simulink library "vco_snn"  (R2023b)
settings: Solver=VariableStepAuto  StartTime=0.0  StopTime=10.0  RelTol=1e-3
libraries: simulink_extras x166, spsSeriesRLCBranchLib x132, spsControlledVoltageSourceLib x126, $bdroot x33, fl_lib x18, msbPllFoundation x10, nesl_utility x9, spsVoltageMeasurementLib x8, simulink x6, spsGroundLib x5, eeGeneralControl x2
(part 1 of 2)
settings Model: Creator=saisanjeet  LastModifiedBy=saisanjeet

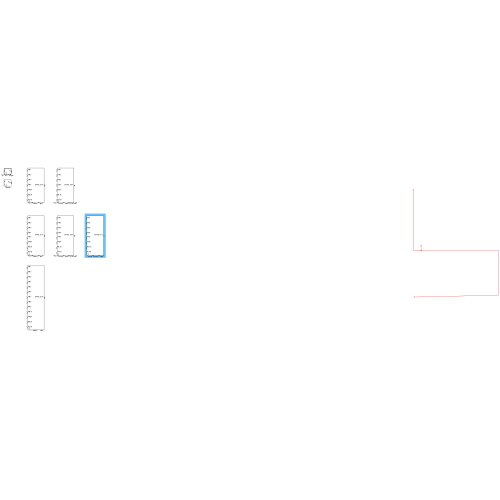
[thumbnail: Simulink's stored preview of the top-level diagram]
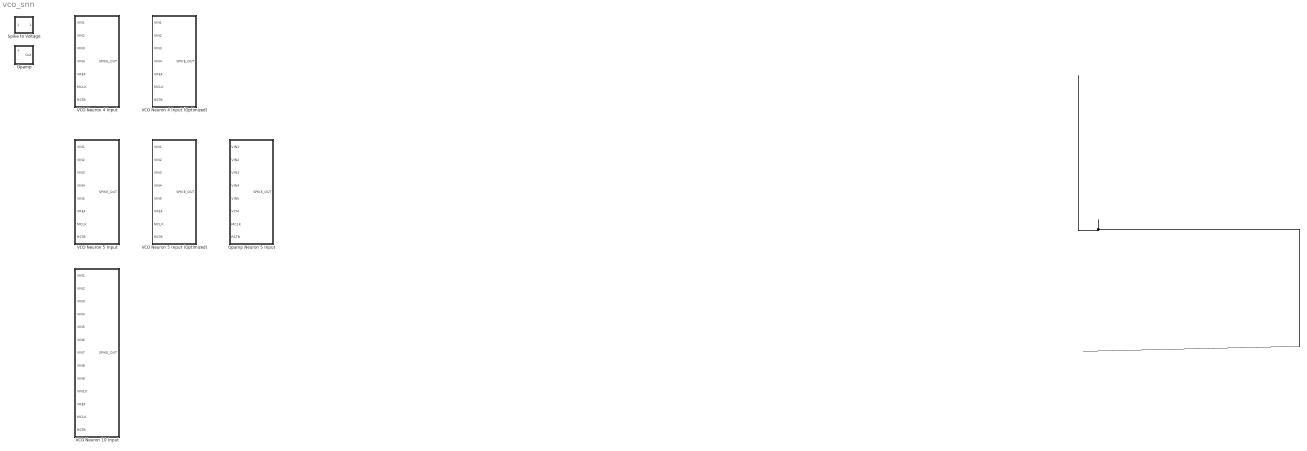
== system vco_snn ==
  Opamp : Subsystem  mask{Gain=1e3}
      mask prompts: Gain "Simulink:blkprm_prompts:GainGain"
      mask TypeOptions Gain: Gain1/Gain
      mask DialogControl Gain Prompt: Gain:
  Opamp Neuron 5 Input : Subsystem  mask{rf=25e3, cf=2e-12, vth=0.45, vcm=0.5, spike_amp=0.2, rin1=25e3, spike_sign1=+1, rin2=25e3, spike_sign2=+1, rin3=25e3, spike_sign3=+1, rin4=25e3, spike_sign4=+1, rin5=25e3, spike_sign5=+1}
      mask prompts: rf "Feedback Resistance (Ohms):"; cf "Feedback Capacitance (F):"; vth "Threshold Voltage (V):"; vcm "Common Mode (V):"; spike_amp "Spike Amplitude (V):"; rin1 "Input 1 Resistance (Ohms):"; spike_sign1 "Input 1 Sign:"; rin2 "Input 2 Resistance (Ohms):"; spike_sign2 "Input 2 Sign:"; rin3 "Input 3 Resistance (Ohms):"; spike_sign3 "Input 3 Sign:"; rin4 "Input 4 Resistance (Ohms):"; spike_sign4 "Input 4 Sign:"; rin5 "Input 5 Resistance (Ohms):"; spike_sign5 "Input 5 Sign:"
      mask TypeOptions rf: Resistor2/R
      mask TypeOptions cf: Capacitor/c
      mask TypeOptions vth:
      | Compare
      | To Constant/const
  Spike to Voltage : Subsystem  TreatAsAtomicUnit=on  mask{vcm=0.5, spike_amp=0.2, sign=+1}
      mask prompts: vcm "Common Mode Voltage (V):"; spike_amp "Spike Amplitude (V):"; sign "Spike Direction:"
      mask TypeOptions vcm: Add Constant/Bias
  VCO Neuron 10 Input : Subsystem  mask{kvco=10e6, center_freq=150e6, xor_res=50e3, vout_cap=1e-12, rf=25000, vth=0.45, vcm=0.5, spike_amp=0.2, rin1=25000, spike_sign1=+1, rin2=25000, spike_sign2=+1, rin3=25000, spike_sign3=+1, rin4=25000, spike_sign4=+1, rin5=25000, spike_sign5=+1, rin6=25000, spike_sign6=+1, rin7=25000, spike_sign7=+1, rin8=25000, spike_sign8=+1, rin9=25000, spike_sign9=+1, rin10=25000, spike_sign10=+1}
      mask prompts: kvco "Kvco (Hz/V):"; center_freq "Center Freq (Hz):"; xor_res "XNOR Resistance (Ohms):"; vout_cap "Output Capacitance (F):"; rf "Feedback Resistance (Ohms):"; vth "Threshold Voltage (V):"; vcm "Input Common Mode (V):"; spike_amp "Spike Amplitude (V):"; rin1 "Input 1 Resistance (Ohms):"; spike_sign1 "Input 1 Sign:"; rin2 "Input 2 Resistance (Ohms):"; spike_sign2 "Input 2 Sign:"; rin3 "Input 3 Resistance (Ohms):"; spike_sign3 "Input 3 Sign:"; rin4 "Input 4 Resistance (Ohms):"; spike_sign4 "Input 4 Sign:"; rin5 "Input 5 Resistance (Ohms):"; spike_sign5 "Input 5 Sign:"; rin6 "Input 6 Resistance (Ohms):"; spike_sign6 "Input 6 Sign:"; rin7 "Input 7 Resistance (Ohms):"; spike_sign7 "Input 7 Sign:"; rin8 "Input 8 Resistance (Ohms):"; spike_sign8 "Input 8 Sign:"; rin9 "Input 9 Resistance (Ohms):"; spike_sign9 "Input 9 Sign:"; rin10 "Input 10 Resistance (Ohms):"; spike_sign10 "Input 10 Sign:"
      mask TypeOptions vout_cap: cout/Capacitance
      mask TypeOptions rf: rf/Resistance
      mask TypeOptions vth: comp/const
  VCO Neuron 4 Input : Subsystem  mask{kvco=10e6, center_freq=150e6, xor_res=50e3, vout_cap=1e-12, rf=25000, vth=0.45, vcm=0.5, spike_amp=0.2, rin1=25000, spike_sign1=+1, rin2=25000, spike_sign2=+1, rin3=25000, spike_sign3=+1, rin4=25000, spike_sign4=+1}
      mask prompts: kvco "Kvco (Hz/V):"; center_freq "Center Freq (Hz):"; xor_res "XNOR Resistance (Ohms):"; vout_cap "Output Capacitance (F):"; rf "Feedback Resistance (Ohms):"; vth "Threshold Voltage (V):"; vcm "Input Common Mode (V):"; spike_amp "Spike Amplitude (V):"; rin1 "Input 1 Resistance (Ohms):"; spike_sign1 "Input 1 Sign:"; rin2 "Input 2 Resistance (Ohms):"; spike_sign2 "Input 2 Sign:"; rin3 "Input 3 Resistance (Ohms):"; spike_sign3 "Input 3 Sign:"; rin4 "Input 4 Resistance (Ohms):"; spike_sign4 "Input 4 Sign:"
      mask TypeOptions vout_cap: cout/Capacitance
      mask TypeOptions rf: rf/Resistance
      mask TypeOptions vth: comp/const
  VCO Neuron 4 Input (Optimized) : Subsystem  mask{kvco=10e6, center_freq=100e6, xor_tau=1.5625e-09, rf=25000, vth=0.45, vcm=0.5, spike_amp=0.2, rin1=25e3, spike_sign1=+1, rin2=25e3, spike_sign2=+1, rin3=25e3, spike_sign3=+1, rin4=25e3, spike_sign4=+1}
      mask prompts: kvco "Kvco (Hz/V):"; center_freq "Center Freq (Hz):"; xor_tau "XNOR Output Time Constant:"; rf "Feedback Resistance (Ohms):"; vth "Threshold Voltage (V):"; vcm "Input Common Mode (V):"; spike_amp "Spike Amplitude (V):"; rin1 "Input 1 Resistance (Ohms):"; spike_sign1 "Input 1 Sign:"; rin2 "Input 2 Resistance (Ohms):"; spike_sign2 "Input 2 Sign:"; rin3 "Input 3 Resistance (Ohms):"; spike_sign3 "Input 3 Sign:"; rin4 "Input 4 Resistance (Ohms):"; spike_sign4 "Input 4 Sign:"
      mask TypeOptions xor_tau: xor_lpf/T
      mask TypeOptions rf: rf/Resistance
      mask TypeOptions vth: comp/const
  VCO Neuron 5 Input : Subsystem  mask{kvco=10e6, center_freq=150e6, xor_res=50e3, vout_cap=1e-12, rf=25000, vth=0.45, vcm=0.5, spike_amp=0.2, rin1=25000, spike_sign1=+1, rin2=25000, spike_sign2=+1, rin3=25000, spike_sign3=+1, rin4=25000, spike_sign4=+1, rin5=25000, spike_sign5=+1}
      mask prompts: kvco "Kvco (Hz/V):"; center_freq "Center Freq (Hz):"; xor_res "XNOR Resistance (Ohms):"; vout_cap "Output Capacitance (F):"; rf "Feedback Resistance (Ohms):"; vth "Threshold Voltage (V):"; vcm "Input Common Mode (V):"; spike_amp "Spike Amplitude (V):"; rin1 "Input 1 Resistance (Ohms):"; spike_sign1 "Input 1 Sign:"; rin2 "Input 2 Resistance (Ohms):"; spike_sign2 "Input 2 Sign:"; rin3 "Input 3 Resistance (Ohms):"; spike_sign3 "Input 3 Sign:"; rin4 "Input 4 Resistance (Ohms):"; spike_sign4 "Input 4 Sign:"; rin5 "Input 5 Resistance (Ohms):"; spike_sign5 "Input 5 Sign:"
      mask TypeOptions vout_cap: cout/Capacitance
      mask TypeOptions rf: rf/Resistance
      mask TypeOptions vth: comp/const
  VCO Neuron 5 Input (Optimized) : Subsystem  mask{kvco=10e6, center_freq=120e6, xor_tau=1.5625e-09, rf=25000, vth=0.45, vcm=0.5, spike_amp=0.2, rin1=25000, spike_sign1=+1, rin2=25000, spike_sign2=+1, rin3=25000, spike_sign3=+1, rin4=25000, spike_sign4=+1, rin5=25000, spike_sign5=+1}
      mask prompts: kvco "Kvco (Hz/V):"; center_freq "Center Freq (Hz):"; xor_tau "XNOR Output Time Constant:"; rf "Feedback Resistance (Ohms):"; vth "Threshold Voltage (V):"; vcm "Input Common Mode (V):"; spike_amp "Spike Amplitude (V):"; rin1 "Input 1 Resistance (Ohms):"; spike_sign1 "Input 1 Sign:"; rin2 "Input 2 Resistance (Ohms):"; spike_sign2 "Input 2 Sign:"; rin3 "Input 3 Resistance (Ohms):"; spike_sign3 "Input 3 Sign:"; rin4 "Input 4 Resistance (Ohms):"; spike_sign4 "Input 4 Sign:"; rin5 "Input 5 Resistance (Ohms):"; spike_sign5 "Input 5 Sign:"
      mask TypeOptions xor_tau: xor_lpf/T
      mask TypeOptions rf: rf/Resistance
      mask TypeOptions vth: comp/const
  connections:
  ?
  ?

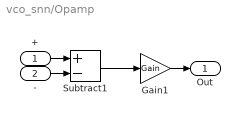
== system vco_snn/Opamp ==
  + : Inport
  - : Inport  Port=2
  Gain1 : Gain  Gain=Gain
  Subtract1 : Sum  Inputs=+-
  Out : Outport
  wires:
  -/1 -> Subtract1/2
  +/1 -> Subtract1/1
  Gain1/1 -> Out/1
  Subtract1/1 -> Gain1/1

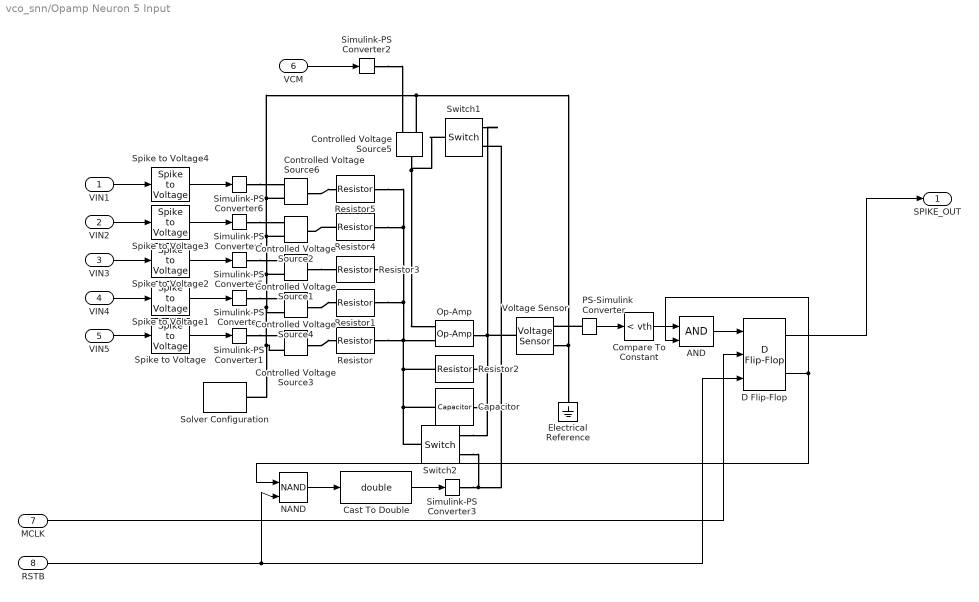
== system vco_snn/Opamp Neuron 5 Input ==
  VIN1 : Inport
  VIN2 : Inport  Port=2
  VIN3 : Inport  Port=3
  VIN4 : Inport  Port=4
  VIN5 : Inport  Port=5
  VCM : Inport  Port=6
  MCLK : Inport  Port=7
  RSTB : Inport  Port=8
  AND : Logic  IconShape=distinctive  AllPortsSameDT=off  OutDataTypeStr=boolean
  Capacitor : fl_lib/Electrical/Electrical Elements/Capacitor  c=cf F  r=1e-6 Ohm  g=0 1/Ohm  i_specify=off  i_priority=None  i=0 A  i_nominal_specify=off  i_nominal_unit=A  i_nominal_value=1  v_specify=on  v_priority=None  v=0 V  v_nominal_specify=off  v_nominal_unit=V  v_nominal_value=1  vc_specify=off  vc_priority=High  vc=0 V  vc_nominal_specify=off  vc_nominal_unit=V  vc_nominal_value=1
  Cast To Double : DataTypeConversion  OutDataTypeStr=double  SaturateOnIntegerOverflow=off  RndMeth=Floor
  Compare To Constant : simulink/Logic and Bit Operations/Compare To Constant  relop=<  const=vth  OutDataTypeStr=boolean
  Controlled Voltage Source{1..6} (6 alike) : fl_lib/Electrical/Electrical Sources/Controlled Voltage Source
  D Flip-Flop : simulink_extras/Flip Flops/D Flip-Flop
  Electrical Reference : fl_lib/Electrical/Electrical Elements/Electrical Reference
  NAND : Logic  Operator=NAND  IconShape=distinctive  AllPortsSameDT=off  OutDataTypeStr=boolean
  Op-Amp : fl_lib/Electrical/Electrical Elements/Op-Amp  outI_specify=off  outI_priority=None  outI=0 A  outI_nominal_specify=off  outI_nominal_unit=A  outI_nominal_value=1
  PS-Simulink Converter : nesl_utility/PS-Simulink Converter  PhysicalDomain=network_engine_domain  SubClassName=ps_output  LeftPortType=input  RightPortType=output  PseudoPeriodic=off  Frequencies=[]  VectorFormat=inherit  Unit=inherit  AffineConversion=off
  Resistor : fl_lib/Electrical/Electrical Elements/Resistor  R=rin5 Ohm  i_specify=off  i_priority=None  i=0 A  i_nominal_specify=off  i_nominal_unit=A  i_nominal_value=1  v_specify=off  v_priority=None  v=0 V  v_nominal_specify=off  v_nominal_unit=V  v_nominal_value=1
  Resistor1 : fl_lib/Electrical/Electrical Elements/Resistor  R=rin4 Ohm  i_specify=off  i_priority=None  i=0 A  i_nominal_specify=off  i_nominal_unit=A  i_nominal_value=1  v_specify=off  v_priority=None  v=0 V  v_nominal_specify=off  v_nominal_unit=V  v_nominal_value=1
  Resistor2 : fl_lib/Electrical/Electrical Elements/Resistor  R=rf Ohm  i_specify=off  i_priority=None  i=0 A  i_nominal_specify=off  i_nominal_unit=A  i_nominal_value=1  v_specify=off  v_priority=None  v=0 V  v_nominal_specify=off  v_nominal_unit=V  v_nominal_value=1
  Resistor3 : fl_lib/Electrical/Electrical Elements/Resistor  R=rin3 Ohm  i_specify=off  i_priority=None  i=0 A  i_nominal_specify=off  i_nominal_unit=A  i_nominal_value=1  v_specify=off  v_priority=None  v=0 V  v_nominal_specify=off  v_nominal_unit=V  v_nominal_value=1
  Resistor4 : fl_lib/Electrical/Electrical Elements/Resistor  R=rin2 Ohm  i_specify=off  i_priority=None  i=0 A  i_nominal_specify=off  i_nominal_unit=A  i_nominal_value=1  v_specify=off  v_priority=None  v=0 V  v_nominal_specify=off  v_nominal_unit=V  v_nominal_value=1
  Resistor5 : fl_lib/Electrical/Electrical Elements/Resistor  R=rin1 Ohm  i_specify=off  i_priority=None  i=0 A  i_nominal_specify=off  i_nominal_unit=A  i_nominal_value=1  v_specify=off  v_priority=None  v=0 V  v_nominal_specify=off  v_nominal_unit=V  v_nominal_value=1
  Simulink-PS Converter{,1..6} (7 alike) : nesl_utility/Simulink-PS Converter  PhysicalDomain=network_engine_domain  SubClassName=ps_input  LeftPortType=input  RightPortType=output  PseudoPeriodic=off  Frequencies=[]  NoiseDistribution=none  NoiseParameters=[]  Unit=1  AffineConversion=off  FilteringAndDerivatives=provide  SimscapeFilterOrder=1  InputFilterTimeConstant=0.001  UdotUserProvided=0
  Solver Configuration : nesl_utility/Solver Configuration  PhysicalDomain=network_engine_domain  SubClassName=solver  LeftPortType=input  RightPortType=generic  Tones=[]  Harmonics=[]  SimulateNoise=off  Profile=off  UseLocalSampling=off  EnableSwitchedLinearOptims=on  FrequencyDomain=off  UseCCode=off  RelTol=0.001  AbsTol=0.001  MinStep=1e-09  ToWorkspace=off  RevertToSquareIcSolve=off  NumHomotopyIterations=100  PhasorMode=off  PhasorModeNumHarmonics=1  ConsistencySolver=NEWTON_XTOL_AFTER_FTOL  IndexReductionMethod=DerivativeReplacement  DoDC=off  ResidualTolerance=1e-09  ConsistencyTolSource=GLOBAL  ConsistencyAbsTol=0.001  ConsistencyRelTol=0.001  ConsistencyTolFactor=0.001  UseLocalSolver=off  LocalSolverChoice=NE_BACKWARD_EULER_ADVANCER  ResolveIndetEquations=on  FunctionEvalNumThread=1  LocalSolverSampleTime=0.001  DoFixedCost=off  MaxNonlinIter=3  MaxModeIter=2  ComputeImpulses=off  ImpulseIterations=2  LinearAlgebra=auto  LinearAlgebraNumThread=0  EquationFormulation=NE_TIME_EF  DelaysMemoryBudget=1024  AutomaticFiltering=on  FilteringTimeConstant=0.001  PartitionStorageMethod=AS_NEEDED  PartitionMemoryBudget=1024  PartitionMethod=ROBUST  MultibodyUseLocalSolver=off  MultibodyLocalSolverChoice=ODE1  MultibodyLocalSolverSampleTime=0.001
  Spike to Voltage : $bdroot/Spike to Voltage  vcm=vcm  spike_amp=spike_amp  sign=spike_sign5
  Spike to Voltage1 : $bdroot/Spike to Voltage  vcm=vcm  spike_amp=spike_amp  sign=spike_sign4
  Spike to Voltage2 : $bdroot/Spike to Voltage  vcm=vcm  spike_amp=spike_amp  sign=spike_sign3
  Spike to Voltage3 : $bdroot/Spike to Voltage  vcm=vcm  spike_amp=spike_amp  sign=spike_sign2
  Spike to Voltage4 : $bdroot/Spike to Voltage  vcm=vcm  spike_amp=spike_amp  sign=spike_sign1
  Switch1 : fl_lib/Electrical/Electrical Elements/Switch  R_closed=0.01 Ohm  G_open=1e-8 1/Ohm  Threshold=0.5  i_specify=off  i_priority=None  i=0 A  i_nominal_specify=off  i_nominal_unit=A  i_nominal_value=1  v_specify=off  v_priority=None  v=0 V  v_nominal_specify=off  v_nominal_unit=V  v_nominal_value=1
  Switch2 : fl_lib/Electrical/Electrical Elements/Switch  R_closed=0.01 Ohm  G_open=1e-8 1/Ohm  Threshold=0.5  i_specify=off  i_priority=None  i=0 A  i_nominal_specify=off  i_nominal_unit=A  i_nominal_value=1  v_specify=off  v_priority=None  v=0 V  v_nominal_specify=off  v_nominal_unit=V  v_nominal_value=1
  Voltage Sensor : fl_lib/Electrical/Electrical Sensors/Voltage Sensor
  SPIKE_OUT : Outport
  wires:
  Compare To Constant/1 -> AND/1
  D Flip-Flop/1 -> SPIKE_OUT/1
  VIN4/1 -> Spike to Voltage1/1
  NAND/1 -> Cast To Double/1
  D Flip-Flop/2 -> NAND/1, AND/2
  RSTB/1 -> NAND/2, D Flip-Flop/3
  MCLK/1 -> D Flip-Flop/2
  PS-Simulink Converter/1 -> Compare To Constant/1
  Cast To Double/1 -> Simulink-PS Converter3/1
  VIN5/1 -> Spike to Voltage/1
  AND/1 -> D Flip-Flop/1
  VCM/1 -> Simulink-PS Converter2/1
  Spike to Voltage/1 -> Simulink-PS Converter1/1
  Spike to Voltage1/1 -> Simulink-PS Converter/1
  Spike to Voltage2/1 -> Simulink-PS Converter5/1
  VIN3/1 -> Spike to Voltage2/1
  VIN2/1 -> Spike to Voltage3/1
  Spike to Voltage3/1 -> Simulink-PS Converter4/1
  Spike to Voltage4/1 -> Simulink-PS Converter6/1
  VIN1/1 -> Spike to Voltage4/1
  connections:
  Simulink-PS Converter1/RConn1 -- Controlled Voltage Source3/RConn1
  PS-Simulink Converter/LConn1 -- Voltage Sensor/RConn1
  Resistor2/LConn1 -- Capacitor/LConn1 -- Switch2/LConn1 -- Op-Amp/LConn2 -- Resistor/RConn1 -- Resistor1/RConn1 -- Resistor3/RConn1 -- Resistor4/RConn1 -- Resistor5/RConn1
  Simulink-PS Converter2/RConn1 -- Controlled Voltage Source5/RConn1
  Controlled Voltage Source4/LConn1 -- Resistor1/LConn1
  Controlled Voltage Source3/LConn1 -- Resistor/LConn1
  Switch1/RConn1 -- Simulink-PS Converter3/RConn1 -- Switch2/RConn1
  Switch1/LConn1 -- Controlled Voltage Source5/LConn1 -- Op-Amp/LConn1
  Op-Amp/RConn1 -- Switch1/RConn2 -- Voltage Sensor/LConn1 -- Resistor2/RConn1 -- Switch2/RConn2 -- Capacitor/RConn1
  Simulink-PS Converter/RConn1 -- Controlled Voltage Source4/RConn1
  Solver Configuration/RConn1 -- Controlled Voltage Source3/RConn2 -- Controlled Voltage Source2/RConn2 -- Voltage Sensor/RConn2 -- Electrical Reference/LConn1 -- Controlled Voltage Source5/RConn2 -- Controlled Voltage Source6/RConn2 -- Controlled Voltage Source1/RConn2 -- Controlled Voltage Source4/RConn2
  Simulink-PS Converter6/RConn1 -- Controlled Voltage Source6/RConn1
  Simulink-PS Converter4/RConn1 -- Controlled Voltage Source2/RConn1
  Simulink-PS Converter5/RConn1 -- Controlled Voltage Source1/RConn1
  Controlled Voltage Source6/LConn1 -- Resistor5/LConn1
  Resistor4/LConn1 -- Controlled Voltage Source2/LConn1
  Controlled Voltage Source1/LConn1 -- Resistor3/LConn1

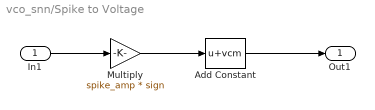
== system vco_snn/Spike to Voltage ==
  In1 : Inport
  Add Constant : Bias  Bias=vcm  SaturateOnIntegerOverflow=off
  Multiply : Gain  Gain=spike_amp * sign
  Out1 : Outport
  wires:
  In1/1 -> Multiply/1
  Add Constant/1 -> Out1/1
  Multiply/1 -> Add Constant/1

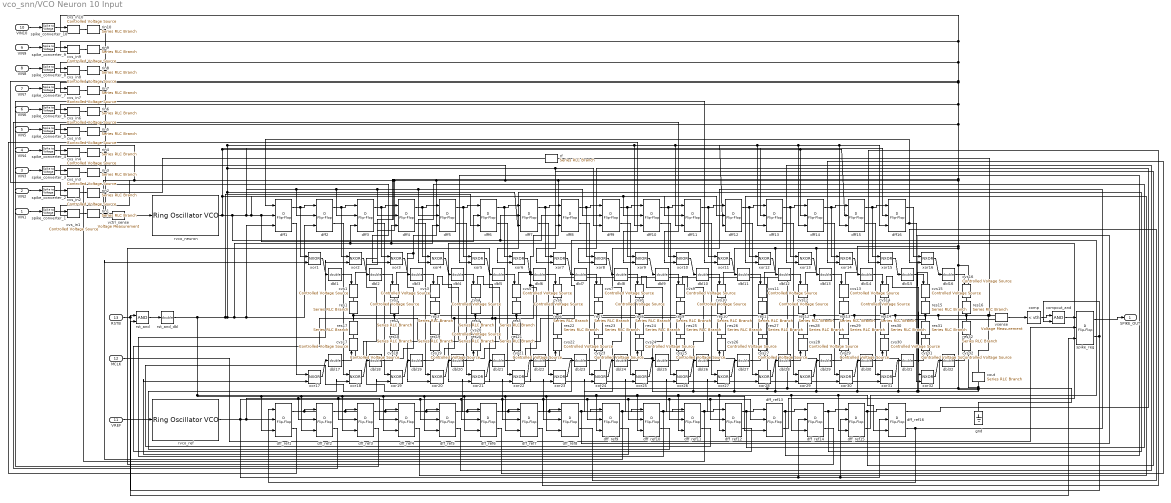
== system vco_snn/VCO Neuron 10 Input ==
  VIN1 : Inport
  VIN2 : Inport  Port=2
  VIN3 : Inport  Port=3
  VIN4 : Inport  Port=4
  VIN5 : Inport  Port=5
  VIN6 : Inport  Port=6
  VIN7 : Inport  Port=7
  VIN8 : Inport  Port=8
  VIN9 : Inport  Port=9
  VIN10 : Inport  Port=10
  VREF : Inport  Port=11
  MCLK : Inport  Port=12
  RSTB : Inport  Port=13
  comp : simulink/Logic and Bit Operations/Compare To Constant  relop=<  const=vth  OutDataTypeStr=boolean
  compout_and : Logic  IconShape=distinctive  AllPortsSameDT=off  OutDataTypeStr=boolean
  cout : spsSeriesRLCBranchLib/Series RLC Branch  LConnTagsString=__new0  RConnTagsString=__new0  BranchType=C  Resistance=1  Inductance=1e-3  SetiL0=off  InitialCurrent=0  Capacitance=vout_cap  Setx0=on  InitialVoltage=0.5  Measurements=None
  cvs{1..32} (32 alike) : spsControlledVoltageSourceLib/Controlled Voltage Source  Initialize=on  Source_Type=AC  Amplitude=0  Phase=0  Frequency=0  Measurements=None
  cvs_in{1..10} (10 alike) : spsControlledVoltageSourceLib/Controlled Voltage Source  Initialize=on  Source_Type=AC  Amplitude=0  Phase=0  Frequency=0  Measurements=None
  dbl{1..32} (32 alike) : DataTypeConversion  OutDataTypeStr=double  SaturateOnIntegerOverflow=off  RndMeth=Floor
  dff{1..16} (16 alike) : simulink_extras/Flip Flops/D Flip-Flop
  dff_ref{1..16} (16 alike) : simulink_extras/Flip Flops/D Flip-Flop
  gnd : spsGroundLib/Ground  LConnTagsString=a
  res{1..32} (32 alike) : spsSeriesRLCBranchLib/Series RLC Branch  LConnTagsString=__new0  RConnTagsString=__new0  BranchType=R  Resistance=xor_res  Inductance=1e-3  SetiL0=off  InitialCurrent=0  Capacitance=1e-6  Setx0=off  InitialVoltage=0  Measurements=None
  rf : spsSeriesRLCBranchLib/Series RLC Branch  LConnTagsString=__new0  RConnTagsString=__new0  BranchType=R  Resistance=rf  Inductance=1e-3  SetiL0=off  InitialCurrent=0  Capacitance=1e-6  Setx0=off  InitialVoltage=0  Measurements=None
  rin1 : spsSeriesRLCBranchLib/Series RLC Branch  LConnTagsString=__new0  RConnTagsString=__new0  BranchType=R  Resistance=rin1  Inductance=1e-3  SetiL0=off  InitialCurrent=0  Capacitance=1e-6  Setx0=off  InitialVoltage=0  Measurements=None
  rin10 : spsSeriesRLCBranchLib/Series RLC Branch  LConnTagsString=__new0  RConnTagsString=__new0  BranchType=R  Resistance=rin10  Inductance=1e-3  SetiL0=off  InitialCurrent=0  Capacitance=1e-6  Setx0=off  InitialVoltage=0  Measurements=None
  rin2 : spsSeriesRLCBranchLib/Series RLC Branch  LConnTagsString=__new0  RConnTagsString=__new0  BranchType=R  Resistance=rin2  Inductance=1e-3  SetiL0=off  InitialCurrent=0  Capacitance=1e-6  Setx0=off  InitialVoltage=0  Measurements=None
  rin3 : spsSeriesRLCBranchLib/Series RLC Branch  LConnTagsString=__new0  RConnTagsString=__new0  BranchType=R  Resistance=rin3  Inductance=1e-3  SetiL0=off  InitialCurrent=0  Capacitance=1e-6  Setx0=off  InitialVoltage=0  Measurements=None
  rin4 : spsSeriesRLCBranchLib/Series RLC Branch  LConnTagsString=__new0  RConnTagsString=__new0  BranchType=R  Resistance=rin4  Inductance=1e-3  SetiL0=off  InitialCurrent=0  Capacitance=1e-6  Setx0=off  InitialVoltage=0  Measurements=None
  rin5 : spsSeriesRLCBranchLib/Series RLC Branch  LConnTagsString=__new0  RConnTagsString=__new0  BranchType=R  Resistance=rin5  Inductance=1e-3  SetiL0=off  InitialCurrent=0  Capacitance=1e-6  Setx0=off  InitialVoltage=0  Measurements=None
  rin6 : spsSeriesRLCBranchLib/Series RLC Branch  LConnTagsString=__new0  RConnTagsString=__new0  BranchType=R  Resistance=rin6  Inductance=1e-3  SetiL0=off  InitialCurrent=0  Capacitance=1e-6  Setx0=off  InitialVoltage=0  Measurements=None
  rin7 : spsSeriesRLCBranchLib/Series RLC Branch  LConnTagsString=__new0  RConnTagsString=__new0  BranchType=R  Resistance=rin7  Inductance=1e-3  SetiL0=off  InitialCurrent=0  Capacitance=1e-6  Setx0=off  InitialVoltage=0  Measurements=None
  rin8 : spsSeriesRLCBranchLib/Series RLC Branch  LConnTagsString=__new0  RConnTagsString=__new0  BranchType=R  Resistance=rin8  Inductance=1e-3  SetiL0=off  InitialCurrent=0  Capacitance=1e-6  Setx0=off  InitialVoltage=0  Measurements=None
  rin9 : spsSeriesRLCBranchLib/Series RLC Branch  LConnTagsString=__new0  RConnTagsString=__new0  BranchType=R  Resistance=rin9  Inductance=1e-3  SetiL0=off  InitialCurrent=0  Capacitance=1e-6  Setx0=off  InitialVoltage=0  Measurements=None
  rst_and : Logic  IconShape=distinctive  AllPortsSameDT=off  OutDataTypeStr=boolean
  rst_and_dbl : DataTypeConversion  OutDataTypeStr=double  SaturateOnIntegerOverflow=off  RndMeth=Floor
  rvco_neuron : msbPllFoundation/Ring Oscillator VCO  SpecifyUsing=Voltage sensitivity  Kvco=kvco*32  Fo=(center_freq - (kvco/2))*32  ControlVoltage=[-5 0 5]  OutputFrequency=[2e9 2.5e9 3e9]  Amplitude=1  ExtraBuffer=off  NBuffer=10  AddPhaseNoise=off  SsbCheck=off  Foffset=[30e3 100e3 1e6 3e6 10e6]  PhaseNoise=[-56 -106 -132 -143 -152]  PeriodJitter=1.7e-15  CornerFrequency=5e5  CustomizeExponent=off  FlickerExponent=1.0  MaxKvco=320000000
  rvco_ref : msbPllFoundation/Ring Oscillator VCO  SpecifyUsing=Voltage sensitivity  Kvco=kvco*32  Fo=(center_freq - (kvco/2))*32  ControlVoltage=[-5 0 5]  OutputFrequency=[2e9 2.5e9 3e9]  Amplitude=1  ExtraBuffer=off  NBuffer=10  AddPhaseNoise=off  SsbCheck=off  Foffset=[30e3 100e3 1e6 3e6 10e6]  PhaseNoise=[-56 -106 -132 -143 -152]  PeriodJitter=1.7e-15  CornerFrequency=5e5  CustomizeExponent=off  FlickerExponent=1.0  MaxKvco=320000000
  spike_converter_1 : $bdroot/Spike to Voltage  vcm=vcm  spike_amp=spike_amp  sign=spike_sign1
  spike_converter_10 : $bdroot/Spike to Voltage  vcm=vcm  spike_amp=spike_amp  sign=spike_sign10
  spike_converter_2 : $bdroot/Spike to Voltage  vcm=vcm  spike_amp=spike_amp  sign=spike_sign2
  spike_converter_3 : $bdroot/Spike to Voltage  vcm=vcm  spike_amp=spike_amp  sign=spike_sign3
  spike_converter_4 : $bdroot/Spike to Voltage  vcm=vcm  spike_amp=spike_amp  sign=spike_sign4
  spike_converter_5 : $bdroot/Spike to Voltage  vcm=vcm  spike_amp=spike_amp  sign=spike_sign5
  spike_converter_6 : $bdroot/Spike to Voltage  vcm=vcm  spike_amp=spike_amp  sign=spike_sign6
  spike_converter_7 : $bdroot/Spike to Voltage  vcm=vcm  spike_amp=spike_amp  sign=spike_sign7
  spike_converter_8 : $bdroot/Spike to Voltage  vcm=vcm  spike_amp=spike_amp  sign=spike_sign8
  spike_converter_9 : $bdroot/Spike to Voltage  vcm=vcm  spike_amp=spike_amp  sign=spike_sign9
  spike_reg : simulink_extras/Flip Flops/D Flip-Flop
  vctrl_sense : spsVoltageMeasurementLib/Voltage Measurement  PhasorSimulation=off  OutputType=Complex  PSBequivalent=0
  vsense : spsVoltageMeasurementLib/Voltage Measurement  PhasorSimulation=off  OutputType=Complex  PSBequivalent=0
  xor{1..32} (32 alike) : Logic  Operator=NXOR  IconShape=distinctive  AllPortsSameDT=off  OutDataTypeStr=boolean
  SPIKE_OUT : Outport
  wires:
  spike_converter_10/1 -> cvs_in10/1
  spike_reg/2 -> compout_and/2, rst_and/2
  MCLK/1 -> spike_reg/2
  dff5/2 -> xor21/1
  dff_ref13/2 -> xor21/2
  dff16/1 -> xor16/1
  VREF/1 -> rvco_ref/1
  rst_and_dbl/1 -> dff_ref8/3, dff_ref13/3, dff_ref7/3, dff_ref6/3, dff_ref5/3, dff_ref4/3, dff_ref3/3, dff_ref2/3, dff_ref1/3, dff_ref15/3, dff_ref16/3, dff_ref14/3, dff_ref12/3, dff_ref11/3, dff_ref10/3, dff_ref9/3, dff1/3, dff2/3, dff4/3, dff5/3, dff3/3, dff8/3, dff9/3, dff11/3, dff12/3, dff10/3, dff15/3, dff16/3, dff14/3, dff13/3, dff7/3, dff6/3
  xor1/1 -> dbl1/1
  xor4/1 -> dbl4/1
  dbl31/1 -> cvs31/1
  dff_ref7/1 -> dff_ref8/1, xor31/2
  VIN5/1 -> spike_converter_5/1
  dff_ref15/1 -> dff_ref16/1, xor7/2
  xor30/1 -> dbl30/1
  spike_converter_9/1 -> cvs_in9/1
  vctrl_sense/1 -> rvco_neuron/1
  xor32/1 -> dbl32/1
  dff14/2 -> xor30/1
  dff1/2 -> xor17/1
  xor29/1 -> dbl29/1
  spike_converter_1/1 -> cvs_in1/1
  comp/1 -> compout_and/1
  xor14/1 -> dbl14/1
  xor8/1 -> dbl8/1
  dff_ref10/2 -> xor18/2
  dff_ref6/2 -> xor14/2
  dff9/1 -> dff10/1, xor9/1
  xor5/1 -> dbl5/1
  dbl8/1 -> cvs8/1
  dff13/2 -> xor29/1
  dbl12/1 -> cvs12/1
  dff_ref6/1 -> dff_ref7/1, xor30/2
  dff_ref7/2 -> xor15/2
  dff15/2 -> xor31/1
  dff_ref9/1 -> dff_ref10/1, xor1/2
  RSTB/1 -> rst_and/1, spike_reg/3
  dff12/1 -> dff13/1, xor12/1
  spike_converter_7/1 -> cvs_in7/1
  dbl11/1 -> cvs11/1
  dbl9/1 -> cvs9/1
  xor21/1 -> dbl21/1
  xor24/1 -> dbl24/1
  dff14/1 -> dff15/1, xor14/1
  dff_ref2/1 -> dff_ref3/1, xor26/2
  xor13/1 -> dbl13/1
  xor16/1 -> dbl16/1
  dbl14/1 -> cvs14/1
  xor31/1 -> dbl31/1
  dff8/2 -> xor24/1
  dff2/1 -> dff3/1, xor2/1
  xor7/1 -> dbl7/1
  xor18/1 -> dbl18/1
  dff11/2 -> xor27/1
  dff_ref3/2 -> xor11/2
  dbl4/1 -> cvs4/1
  dff_ref5/1 -> dff_ref6/1, xor29/2
  spike_reg/1 -> SPIKE_OUT/1
  dbl32/1 -> cvs32/1
  compout_and/1 -> spike_reg/1
  dbl13/1 -> cvs13/1
  dff6/1 -> dff7/1, xor6/1
  dbl21/1 -> cvs21/1
  dbl18/1 -> cvs18/1
  dbl29/1 -> cvs29/1
  dbl7/1 -> cvs7/1
  xor28/1 -> dbl28/1
  dbl23/1 -> cvs23/1
  dff_ref4/2 -> xor12/2
  dff12/2 -> xor28/1
  dff_ref8/2 -> xor16/2
  dbl16/1 -> cvs16/1
  dbl5/1 -> cvs5/1
  dbl10/1 -> cvs10/1
  VIN4/1 -> spike_converter_4/1
  xor2/1 -> dbl2/1
  xor11/1 -> dbl11/1
  spike_converter_6/1 -> cvs_in6/1
  dbl6/1 -> cvs6/1
  dff3/2 -> xor19/1
  dff6/2 -> xor22/1
  dbl2/1 -> cvs2/1
  xor3/1 -> dbl3/1
  dff_ref13/1 -> dff_ref14/1, xor5/2
  dff_ref2/2 -> xor10/2
  dbl17/1 -> cvs17/1
  dff8/1 -> dff9/1, xor8/1
  dff9/2 -> xor25/1
  VIN2/1 -> spike_converter_2/1
  dbl1/1 -> cvs1/1
  dbl30/1 -> cvs30/1
  spike_converter_3/1 -> cvs_in3/1
  xor10/1 -> dbl10/1
  VIN10/1 -> spike_converter_10/1
  dff_ref1/2 -> xor9/2
  xor25/1 -> dbl25/1
  spike_converter_5/1 -> cvs_in5/1
  dff_ref16/2 -> dff_ref1/1, xor24/2
  dff11/1 -> dff12/1, xor11/1
  dbl20/1 -> cvs20/1
  VIN3/1 -> spike_converter_3/1
  vsense/1 -> comp/1
  dbl24/1 -> cvs24/1
  dff10/2 -> xor26/1
  dff_ref11/2 -> xor19/2
  dff_ref5/2 -> xor13/2
  dff_ref10/1 -> dff_ref11/1, xor2/2
  dff4/1 -> dff5/1, xor4/1
  dbl27/1 -> cvs27/1
  rst_and/1 -> rst_and_dbl/1
  dff7/1 -> dff8/1, xor7/1
  xor23/1 -> dbl23/1
  dff_ref9/2 -> xor17/2
  dff_ref8/1 -> dff_ref9/1, xor32/2
  VIN6/1 -> spike_converter_6/1
  VIN8/1 -> spike_converter_8/1
  dff3/1 -> dff4/1, xor3/1
  dff_ref12/1 -> dff_ref13/1, xor4/2
  dff5/1 -> dff6/1, xor5/1
  dff1/1 -> dff2/1, xor1/1
  dff_ref11/1 -> dff_ref12/1, xor3/2
  xor27/1 -> dbl27/1
  VIN9/1 -> spike_converter_9/1
  dff_ref4/1 -> dff_ref5/1, xor28/2
  dff13/1 -> dff14/1, xor13/1
  dff4/2 -> xor20/1
  spike_converter_8/1 -> cvs_in8/1
  xor6/1 -> dbl6/1
  xor17/1 -> dbl17/1
  dbl25/1 -> cvs25/1
  dbl26/1 -> cvs26/1
  dbl3/1 -> cvs3/1
  xor9/1 -> dbl9/1
  dbl22/1 -> cvs22/1
  dff10/1 -> dff11/1, xor10/1
  xor19/1 -> dbl19/1
  dff_ref15/2 -> xor23/2
  dff_ref12/2 -> xor20/2
  rvco_ref/1 -> dff_ref15/2, dff_ref16/2, dff_ref14/2, dff_ref3/2, dff_ref4/2, dff_ref2/2, dff_ref1/2, dff_ref12/2, dff_ref13/2, dff_ref11/2, dff_ref10/2, dff_ref9/2, dff_ref8/2, dff_ref7/2, dff_ref6/2, dff_ref5/2
  dff15/1 -> dff16/1, xor15/1
  dff_ref3/1 -> dff_ref4/1, xor27/2
  xor22/1 -> dbl22/1
  dff_ref14/2 -> xor22/2
  dff2/2 -> xor18/1
  dbl19/1 -> cvs19/1
  dff16/2 -> dff1/1, xor32/1
  rvco_neuron/1 -> dff7/2, dff8/2, dff1/2, dff6/2, dff12/2, dff5/2, dff9/2, dff4/2, dff3/2, dff2/2, dff16/2, dff10/2, dff11/2, dff14/2, dff15/2, dff13/2
  dbl28/1 -> cvs28/1
  dff_ref1/1 -> dff_ref2/1, xor25/2
  VIN1/1 -> spike_converter_1/1
  dff_ref14/1 -> dff_ref15/1, xor6/2
  xor12/1 -> dbl12/1
  VIN7/1 -> spike_converter_7/1
  spike_converter_2/1 -> cvs_in2/1
  xor20/1 -> dbl20/1
  xor15/1 -> dbl15/1
  dff7/2 -> xor23/1
  spike_converter_4/1 -> cvs_in4/1
  dbl15/1 -> cvs15/1
  dff_ref16/1 -> xor8/2
  xor26/1 -> dbl26/1
  connections:
  cvs_in10/RConn1 -- rin10/LConn1
  cvs26/RConn1 -- res26/RConn1
  cvs29/RConn1 -- res29/RConn1
  cvs18/RConn1 -- res18/RConn1
  cvs19/RConn1 -- res19/RConn1
  cvs32/RConn1 -- res32/RConn1
  cvs_in5/RConn1 -- rin5/LConn1
  rin1/RConn1 -- vctrl_sense/LConn1 -- rin2/RConn1 -- rf/LConn1 -- rin3/RConn1 -- rin4/RConn1 -- rin5/RConn1 -- rin6/RConn1 -- rin7/RConn1 -- rin8/RConn1 -- rin10/RConn1 -- rin9/RConn1
  cvs_in1/RConn1 -- rin1/LConn1
  cvs_in7/RConn1 -- rin7/LConn1
  cvs12/RConn1 -- res12/RConn1
  cvs_in2/RConn1 -- rin2/LConn1
  cvs21/RConn1 -- res21/RConn1
  cvs15/RConn1 -- res15/RConn1
  cvs31/RConn1 -- res31/RConn1
  cvs11/RConn1 -- res11/RConn1
  cvs27/RConn1 -- res27/RConn1
  cvs_in8/RConn1 -- rin8/LConn1
  cvs25/RConn1 -- res25/RConn1
  cvs4/RConn1 -- res4/RConn1
  cvs17/RConn1 -- res17/RConn1
  cvs2/RConn1 -- res2/RConn1
  cvs20/RConn1 -- res20/RConn1
  cvs10/RConn1 -- res10/RConn1
  cvs7/RConn1 -- res7/RConn1
  cvs_in3/RConn1 -- rin3/LConn1
  cvs1/RConn1 -- res1/RConn1
  cvs3/RConn1 -- res3/RConn1
  cvs22/RConn1 -- res22/RConn1
  cvs_in4/RConn1 -- rin4/LConn1
  cvs13/RConn1 -- res13/RConn1
  cvs5/RConn1 -- res5/RConn1
  cvs28/RConn1 -- res28/RConn1
  cvs16/RConn1 -- res16/RConn1
  cvs14/RConn1 -- res14/RConn1
  cvs6/RConn1 -- res6/RConn1
  cvs30/RConn1 -- res30/RConn1
  cvs_in9/RConn1 -- rin9/LConn1
  cvs8/RConn1 -- res8/RConn1
  cvs23/RConn1 -- res23/RConn1
  cvs24/RConn1 -- res24/RConn1
  cvs_in6/RConn1 -- rin6/LConn1
  cvs18/LConn1 -- cvs2/LConn1 -- cvs17/LConn1 -- vctrl_sense/LConn2 -- cvs1/LConn1 -- cvs_in10/LConn1 -- cvs_in9/LConn1 -- cvs_in8/LConn1 -- cvs_in2/LConn1 -- cvs_in7/LConn1 -- cvs_in6/LConn1 -- cvs_in5/LConn1 -- cvs22/LConn1 -- cvs_in4/LConn1 -- cvs_in1/LConn1 -- cvs_in3/LConn1 -- cvs11/LConn1 -- cvs10/LConn1 -- cvs12/LConn1 -- cvs24/LConn1 -- cvs8/LConn1 -- cvs25/LConn1 -- cvs9/LConn1 -- cvs26/LConn1 -- cvs27/LConn1 -- cvs28/LConn1 -- cvs29/LConn1 -- cvs30/LConn1 -- cvs15/LConn1 -- cvs14/LConn1 -- vsense/LConn2 -- cvs23/LConn1 -- cvs6/LConn1 -- cvs7/LConn1 -- cout/RConn1 -- cvs32/LConn1 -- gnd/LConn1 -- cvs31/LConn1 -- cvs16/LConn1 -- cvs13/LConn1 -- cvs5/LConn1 -- cvs21/LConn1 -- cvs20/LConn1 -- cvs4/LConn1 -- cvs19/LConn1 -- cvs3/LConn1
  cvs9/RConn1 -- res9/RConn1
  res8/LConn1 -- res7/LConn1 -- res9/LConn1 -- res1/LConn1 -- res17/LConn1 -- res18/LConn1 -- res2/LConn1 -- res19/LConn1 -- res3/LConn1 -- res20/LConn1 -- res4/LConn1 -- res21/LConn1 -- res5/LConn1 -- res22/LConn1 -- res6/LConn1 -- res23/LConn1 -- res24/LConn1 -- res25/LConn1 -- res26/LConn1 -- res10/LConn1 -- res27/LConn1 -- res11/LConn1 -- res28/LConn1 -- res12/LConn1 -- res13/LConn1 -- res29/LConn1 -- res14/LConn1 -- res30/LConn1 -- res15/LConn1 -- res31/LConn1 -- res16/LConn1 -- res32/LConn1 -- cout/LConn1 -- rf/RConn1 -- vsense/LConn1

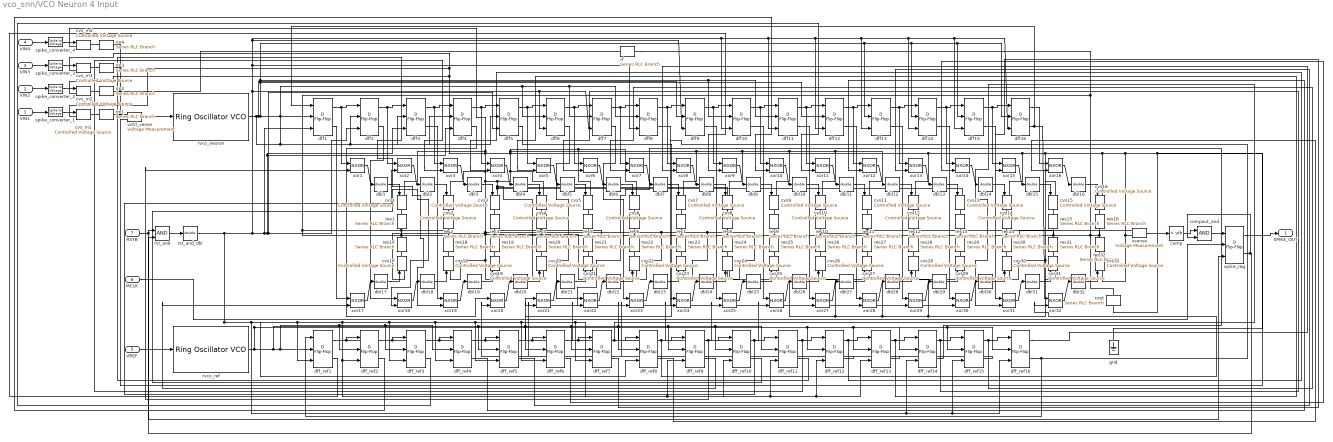
== system vco_snn/VCO Neuron 4 Input ==
  VIN1 : Inport
  VIN2 : Inport  Port=2
  VIN3 : Inport  Port=3
  VIN4 : Inport  Port=4
  VREF : Inport  Port=5
  MCLK : Inport  Port=6
  RSTB : Inport  Port=7
  comp : simulink/Logic and Bit Operations/Compare To Constant  relop=<  const=vth  OutDataTypeStr=boolean
  compout_and : Logic  IconShape=distinctive  AllPortsSameDT=off  OutDataTypeStr=boolean
  cout : spsSeriesRLCBranchLib/Series RLC Branch  LConnTagsString=__new0  RConnTagsString=__new0  BranchType=C  Resistance=1  Inductance=1e-3  SetiL0=off  InitialCurrent=0  Capacitance=vout_cap  Setx0=on  InitialVoltage=0.5  Measurements=None
  cvs{1..32} (32 alike) : spsControlledVoltageSourceLib/Controlled Voltage Source  Initialize=on  Source_Type=AC  Amplitude=0  Phase=0  Frequency=0  Measurements=None
  cvs_in{1..4} (4 alike) : spsControlledVoltageSourceLib/Controlled Voltage Source  Initialize=on  Source_Type=AC  Amplitude=0  Phase=0  Frequency=0  Measurements=None
  dbl{1..32} (32 alike) : DataTypeConversion  OutDataTypeStr=double  SaturateOnIntegerOverflow=off  RndMeth=Floor
  dff{1..16} (16 alike) : simulink_extras/Flip Flops/D Flip-Flop
  dff_ref{1..16} (16 alike) : simulink_extras/Flip Flops/D Flip-Flop
  gnd : spsGroundLib/Ground  LConnTagsString=a
  res{1..32} (32 alike) : spsSeriesRLCBranchLib/Series RLC Branch  LConnTagsString=__new0  RConnTagsString=__new0  BranchType=R  Resistance=xor_res  Inductance=1e-3  SetiL0=off  InitialCurrent=0  Capacitance=1e-6  Setx0=off  InitialVoltage=0  Measurements=None
  rf : spsSeriesRLCBranchLib/Series RLC Branch  LConnTagsString=__new0  RConnTagsString=__new0  BranchType=R  Resistance=rf  Inductance=1e-3  SetiL0=off  InitialCurrent=0  Capacitance=1e-6  Setx0=off  InitialVoltage=0  Measurements=None
  rin1 : spsSeriesRLCBranchLib/Series RLC Branch  LConnTagsString=__new0  RConnTagsString=__new0  BranchType=R  Resistance=rin1  Inductance=1e-3  SetiL0=off  InitialCurrent=0  Capacitance=1e-6  Setx0=off  InitialVoltage=0  Measurements=None
  rin2 : spsSeriesRLCBranchLib/Series RLC Branch  LConnTagsString=__new0  RConnTagsString=__new0  BranchType=R  Resistance=rin2  Inductance=1e-3  SetiL0=off  InitialCurrent=0  Capacitance=1e-6  Setx0=off  InitialVoltage=0  Measurements=None
  rin3 : spsSeriesRLCBranchLib/Series RLC Branch  LConnTagsString=__new0  RConnTagsString=__new0  BranchType=R  Resistance=rin3  Inductance=1e-3  SetiL0=off  InitialCurrent=0  Capacitance=1e-6  Setx0=off  InitialVoltage=0  Measurements=None
  rin4 : spsSeriesRLCBranchLib/Series RLC Branch  LConnTagsString=__new0  RConnTagsString=__new0  BranchType=R  Resistance=rin4  Inductance=1e-3  SetiL0=off  InitialCurrent=0  Capacitance=1e-6  Setx0=off  InitialVoltage=0  Measurements=None
  rst_and : Logic  IconShape=distinctive  AllPortsSameDT=off  OutDataTypeStr=boolean
  rst_and_dbl : DataTypeConversion  OutDataTypeStr=double  SaturateOnIntegerOverflow=off  RndMeth=Floor
  rvco_neuron : msbPllFoundation/Ring Oscillator VCO  SpecifyUsing=Voltage sensitivity  Kvco=kvco*32  Fo=(center_freq - (kvco/2))*32  ControlVoltage=[-5 0 5]  OutputFrequency=[2e9 2.5e9 3e9]  Amplitude=1  ExtraBuffer=off  NBuffer=10  AddPhaseNoise=off  SsbCheck=off  Foffset=[30e3 100e3 1e6 3e6 10e6]  PhaseNoise=[-56 -106 -132 -143 -152]  PeriodJitter=1.7e-15  CornerFrequency=5e5  CustomizeExponent=off  FlickerExponent=1.0  MaxKvco=320000000
  rvco_ref : msbPllFoundation/Ring Oscillator VCO  SpecifyUsing=Voltage sensitivity  Kvco=kvco*32  Fo=(center_freq - (kvco/2))*32  ControlVoltage=[-5 0 5]  OutputFrequency=[2e9 2.5e9 3e9]  Amplitude=1  ExtraBuffer=off  NBuffer=10  AddPhaseNoise=off  SsbCheck=off  Foffset=[30e3 100e3 1e6 3e6 10e6]  PhaseNoise=[-56 -106 -132 -143 -152]  PeriodJitter=1.7e-15  CornerFrequency=5e5  CustomizeExponent=off  FlickerExponent=1.0  MaxKvco=320000000
  spike_converter_1 : $bdroot/Spike to Voltage  vcm=vcm  spike_amp=spike_amp  sign=spike_sign1
  spike_converter_2 : $bdroot/Spike to Voltage  vcm=vcm  spike_amp=spike_amp  sign=spike_sign2
  spike_converter_3 : $bdroot/Spike to Voltage  vcm=vcm  spike_amp=spike_amp  sign=spike_sign3
  spike_converter_4 : $bdroot/Spike to Voltage  vcm=vcm  spike_amp=spike_amp  sign=spike_sign4
  spike_reg : simulink_extras/Flip Flops/D Flip-Flop
  vctrl_sense : spsVoltageMeasurementLib/Voltage Measurement  PhasorSimulation=off  OutputType=Complex  PSBequivalent=0
  vsense : spsVoltageMeasurementLib/Voltage Measurement  PhasorSimulation=off  OutputType=Complex  PSBequivalent=0
  xor{1..32} (32 alike) : Logic  Operator=NXOR  IconShape=distinctive  AllPortsSameDT=off  OutDataTypeStr=boolean
  SPIKE_OUT : Outport
  wires:
  dff15/2 -> xor31/1
  vsense/1 -> comp/1
  dbl2/1 -> cvs2/1
  VREF/1 -> rvco_ref/1
  dbl28/1 -> cvs28/1
  xor24/1 -> dbl24/1
  dff_ref14/2 -> xor22/2
  dbl16/1 -> cvs16/1
  dbl18/1 -> cvs18/1
  spike_converter_1/1 -> cvs_in1/1
  xor26/1 -> dbl26/1
  dbl17/1 -> cvs17/1
  xor16/1 -> dbl16/1
  dff_ref2/2 -> xor10/2
  dff_ref10/2 -> xor18/2
  dff3/2 -> xor19/1
  dff_ref13/2 -> xor21/2
  xor10/1 -> dbl10/1
  dbl5/1 -> cvs5/1
  dff5/2 -> xor21/1
  dff10/2 -> xor26/1
  dbl9/1 -> cvs9/1
  dff_ref6/1 -> dff_ref7/1, xor30/2
  dbl13/1 -> cvs13/1
  dff_ref6/2 -> xor14/2
  dff11/2 -> xor27/1
  xor12/1 -> dbl12/1
  dbl25/1 -> cvs25/1
  dff14/1 -> dff15/1, xor14/1
  dbl30/1 -> cvs30/1
  dff_ref8/2 -> xor16/2
  dff13/2 -> xor29/1
  xor28/1 -> dbl28/1
  dbl4/1 -> cvs4/1
  dff4/2 -> xor20/1
  dbl22/1 -> cvs22/1
  dbl29/1 -> cvs29/1
  dbl11/1 -> cvs11/1
  dff_ref3/2 -> xor11/2
  dbl32/1 -> cvs32/1
  dff_ref7/1 -> dff_ref8/1, xor31/2
  xor1/1 -> dbl1/1
  comp/1 -> compout_and/1
  xor8/1 -> dbl8/1
  dff_ref12/2 -> xor20/2
  dbl1/1 -> cvs1/1
  dff_ref15/2 -> xor23/2
  xor29/1 -> dbl29/1
  dbl7/1 -> cvs7/1
  dff11/1 -> dff12/1, xor11/1
  xor5/1 -> dbl5/1
  dff_ref3/1 -> dff_ref4/1, xor27/2
  dbl21/1 -> cvs21/1
  dff9/2 -> xor25/1
  dbl20/1 -> cvs20/1
  dff12/1 -> dff13/1, xor12/1
  VIN4/1 -> spike_converter_4/1
  dbl19/1 -> cvs19/1
  xor23/1 -> dbl23/1
  xor22/1 -> dbl22/1
  dbl12/1 -> cvs12/1
  xor11/1 -> dbl11/1
  dff_ref1/1 -> dff_ref2/1, xor25/2
  dbl14/1 -> cvs14/1
  dff1/1 -> dff2/1, xor1/1
  MCLK/1 -> spike_reg/2
  dff_ref9/1 -> dff_ref10/1, xor1/2
  RSTB/1 -> rst_and/1, spike_reg/3
  dff2/1 -> dff3/1, xor2/1
  dff_ref5/2 -> xor13/2
  compout_and/1 -> spike_reg/1
  dff_ref9/2 -> xor17/2
  xor18/1 -> dbl18/1
  dff10/1 -> dff11/1, xor10/1
  dff_ref1/2 -> xor9/2
  spike_reg/1 -> SPIKE_OUT/1
  dbl27/1 -> cvs27/1
  xor6/1 -> dbl6/1
  dff_ref13/1 -> dff_ref14/1, xor5/2
  dff2/2 -> xor18/1
  dff_ref10/1 -> dff_ref11/1, xor2/2
  dff3/1 -> dff4/1, xor3/1
  dbl26/1 -> cvs26/1
  xor31/1 -> dbl31/1
  dff4/1 -> dff5/1, xor4/1
  spike_converter_2/1 -> cvs_in2/1
  dff13/1 -> dff14/1, xor13/1
  dff5/1 -> dff6/1, xor5/1
  xor19/1 -> dbl19/1
  xor25/1 -> dbl25/1
  xor3/1 -> dbl3/1
  dbl23/1 -> cvs23/1
  VIN2/1 -> spike_converter_2/1
  rst_and_dbl/1 -> dff_ref15/3, dff_ref16/3, dff_ref14/3, dff_ref8/3, dff_ref12/3, dff_ref13/3, dff_ref11/3, dff_ref2/3, dff_ref9/3, dff_ref10/3, dff_ref7/3, dff_ref6/3, dff_ref5/3, dff_ref4/3, dff_ref3/3, dff_ref1/3, dff2/3, dff5/3, dff3/3, dff4/3, dff1/3, dff6/3, dff7/3, dff15/3, dff16/3, dff14/3, dff13/3, dff12/3, dff11/3, dff10/3, dff9/3, dff8/3
  dff7/2 -> xor23/1
  dff14/2 -> xor30/1
  dbl8/1 -> cvs8/1
  dff_ref4/1 -> dff_ref5/1, xor28/2
  xor21/1 -> dbl21/1
  dff_ref16/2 -> dff_ref1/1, xor24/2
  xor2/1 -> dbl2/1
  dff_ref5/1 -> dff_ref6/1, xor29/2
  xor4/1 -> dbl4/1
  dff12/2 -> xor28/1
  xor7/1 -> dbl7/1
  dff_ref16/1 -> xor8/2
  spike_converter_3/1 -> cvs_in3/1
  dff1/2 -> xor17/1
  dff_ref11/1 -> dff_ref12/1, xor3/2
  rvco_ref/1 -> dff_ref3/2, dff_ref4/2, dff_ref2/2, dff_ref1/2, dff_ref10/2, dff_ref11/2, dff_ref9/2, dff_ref8/2, dff_ref7/2, dff_ref6/2, dff_ref5/2, dff_ref15/2, dff_ref16/2, dff_ref13/2, dff_ref14/2, dff_ref12/2
  dbl15/1 -> cvs15/1
  dff9/1 -> dff10/1, xor9/1
  dff_ref4/2 -> xor12/2
  dff15/1 -> dff16/1, xor15/1
  VIN3/1 -> spike_converter_3/1
  dff16/2 -> dff1/1, xor32/1
  dbl31/1 -> cvs31/1
  dff_ref8/1 -> dff_ref9/1, xor32/2
  dff_ref14/1 -> dff_ref15/1, xor6/2
  dff_ref15/1 -> dff_ref16/1, xor7/2
  dff_ref11/2 -> xor19/2
  dbl24/1 -> cvs24/1
  dff8/2 -> xor24/1
  xor17/1 -> dbl17/1
  xor13/1 -> dbl13/1
  rvco_neuron/1 -> dff2/2, dff3/2, dff4/2, dff7/2, dff8/2, dff6/2, dff1/2, dff10/2, dff11/2, dff15/2, dff16/2, dff14/2, dff13/2, dff12/2, dff9/2, dff5/2
  dbl10/1 -> cvs10/1
  xor14/1 -> dbl14/1
  dff8/1 -> dff9/1, xor8/1
  xor27/1 -> dbl27/1
  xor30/1 -> dbl30/1
  dbl3/1 -> cvs3/1
  dff7/1 -> dff8/1, xor7/1
  xor32/1 -> dbl32/1
  VIN1/1 -> spike_converter_1/1
  rst_and/1 -> rst_and_dbl/1
  dff6/1 -> dff7/1, xor6/1
  spike_reg/2 -> compout_and/2, rst_and/2
  xor15/1 -> dbl15/1
  dff6/2 -> xor22/1
  spike_converter_4/1 -> cvs_in4/1
  dbl6/1 -> cvs6/1
  xor9/1 -> dbl9/1
  xor20/1 -> dbl20/1
  dff_ref12/1 -> dff_ref13/1, xor4/2
  dff_ref7/2 -> xor15/2
  dff16/1 -> xor16/1
  dff_ref2/1 -> dff_ref3/1, xor26/2
  vctrl_sense/1 -> rvco_neuron/1
  connections:
  cvs31/RConn1 -- res31/RConn1
  cvs_in3/RConn1 -- rin3/LConn1
  cvs8/RConn1 -- res8/RConn1
  cvs_in4/RConn1 -- rin4/LConn1
  cvs22/RConn1 -- res22/RConn1
  cvs5/RConn1 -- res5/RConn1
  cvs6/RConn1 -- res6/RConn1
  cvs28/RConn1 -- res28/RConn1
  cvs27/RConn1 -- res27/RConn1
  cvs9/RConn1 -- res9/RConn1
  cvs14/RConn1 -- res14/RConn1
  cvs10/RConn1 -- res10/RConn1
  cvs19/RConn1 -- res19/RConn1
  cvs7/RConn1 -- res7/RConn1
  cvs21/RConn1 -- res21/RConn1
  cvs30/RConn1 -- res30/RConn1
  cvs4/RConn1 -- res4/RConn1
  cvs25/RConn1 -- res25/RConn1
  cvs3/RConn1 -- res3/RConn1
  cvs_in2/RConn1 -- rin2/LConn1
  cvs29/RConn1 -- res29/RConn1
  cvs1/RConn1 -- res1/RConn1
  cvs24/RConn1 -- res24/RConn1
  cvs_in1/RConn1 -- rin1/LConn1
  cvs18/RConn1 -- res18/RConn1
  cvs13/RConn1 -- res13/RConn1
  cvs12/RConn1 -- res12/RConn1
  res18/LConn1 -- res17/LConn1 -- res32/LConn1 -- res16/LConn1 -- res20/LConn1 -- res19/LConn1 -- res4/LConn1 -- res3/LConn1 -- res21/LConn1 -- res5/LConn1 -- res22/LConn1 -- res6/LConn1 -- res23/LConn1 -- res7/LConn1 -- res24/LConn1 -- res8/LConn1 -- res25/LConn1 -- res9/LConn1 -- res10/LConn1 -- res27/LConn1 -- vsense/LConn1 -- res26/LConn1 -- res11/LConn1 -- res28/LConn1 -- res12/LConn1 -- res29/LConn1 -- res13/LConn1 -- res30/LConn1 -- res14/LConn1 -- res31/LConn1 -- res15/LConn1 -- cout/LConn1 -- rf/RConn1 -- res2/LConn1 -- res1/LConn1
  cvs26/RConn1 -- res26/RConn1
  cvs2/RConn1 -- res2/RConn1
  cvs11/RConn1 -- res11/RConn1
  cvs20/RConn1 -- res20/RConn1
  cvs32/RConn1 -- res32/RConn1
  cvs15/RConn1 -- res15/RConn1
  cvs23/RConn1 -- res23/RConn1
  rin4/RConn1 -- rin3/RConn1 -- rin2/RConn1 -- rf/LConn1 -- rin1/RConn1 -- vctrl_sense/LConn1
  cout/RConn1 -- gnd/LConn1 -- cvs6/LConn1 -- cvs5/LConn1 -- cvs11/LConn1 -- cvs10/LConn1 -- cvs9/LConn1 -- cvs8/LConn1 -- cvs7/LConn1 -- cvs19/LConn1 -- cvs18/LConn1 -- cvs21/LConn1 -- cvs17/LConn1 -- cvs24/LConn1 -- cvs23/LConn1 -- cvs22/LConn1 -- cvs_in3/LConn1 -- cvs_in1/LConn1 -- cvs_in2/LConn1 -- cvs26/LConn1 -- cvs25/LConn1 -- cvs27/LConn1 -- cvs28/LConn1 -- cvs30/LConn1 -- vctrl_sense/LConn2 -- cvs_in4/LConn1 -- cvs1/LConn1 -- cvs2/LConn1 -- cvs13/LConn1 -- cvs3/LConn1 -- cvs29/LConn1 -- cvs20/LConn1 -- cvs4/LConn1 -- cvs12/LConn1 -- cvs14/LConn1 -- cvs31/LConn1 -- cvs15/LConn1 -- cvs16/LConn1 -- cvs32/LConn1 -- vsense/LConn2
  cvs16/RConn1 -- res16/RConn1
  cvs17/RConn1 -- res17/RConn1
